simulink model "faza"  (R2025b)
settings: Solver=VariableStepAuto  StartTime=0.0  StopTime=100  MaxStep=0.01  RelTol=1e-3
values from neighbouring files (symbols this model uses):
  czas_skoku = 10    [portrety_fazowe.m]
  ksi = -5    [portrety_fazowe.m]
  omega = 2    [portrety_fazowe.m]
  skok = 0    [portrety_fazowe.m]
  x10 = tabx10(i)    [portrety_fazowe.m]
  x20 = tabx20(i)    [portrety_fazowe.m]
settings Model: Creator=mikol  LastModifiedBy=mikol

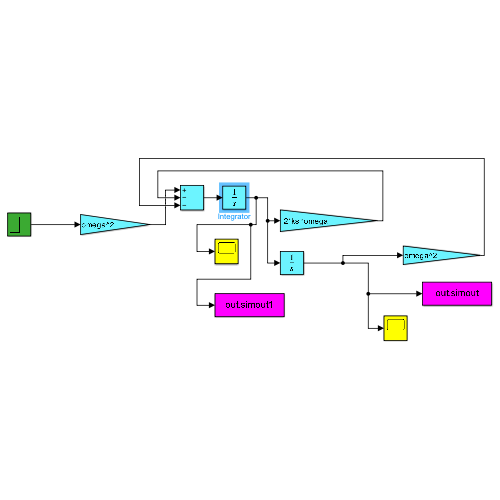
[thumbnail: Simulink's stored preview of the top-level diagram]
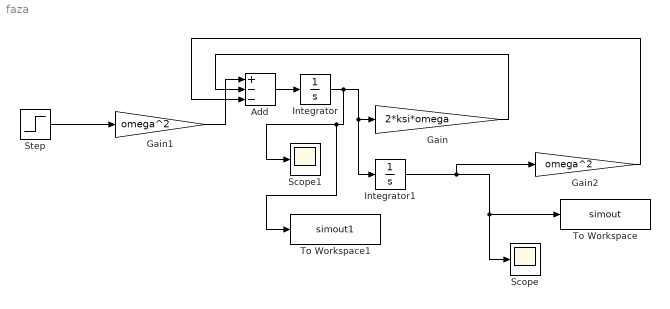
== system faza ==
  Add : Sum  Inputs=+--
  Gain : Gain  Gain=2*ksi*omega
  Gain1 : Gain  Gain=omega^2
  Gain2 : Gain  Gain=omega^2
  Integrator : Integrator  InitialCondition=x10
  Integrator1 : Integrator  InitialCondition=x20
  Scope : Scope
      settings: ActiveDisplayYMinimum=-1  ActiveDisplayYMaximum=1
  Scope1 : Scope
      settings: ActiveDisplayYMinimum=-1  ActiveDisplayYMaximum=1
  Step : Step  Time=czas_skoku  After=skok  SampleTime=0
  To Workspace : ToWorkspace  VariableName=simout  SampleTime=-1
  To Workspace1 : ToWorkspace  VariableName=simout1  SampleTime=-1
  wires:
  Integrator/1 -> To Workspace1/1, Scope1/1, Gain/1, Integrator1/1
  Integrator1/1 -> Scope/1, To Workspace/1, Gain2/1
  Step/1 -> Gain1/1
  Gain1/1 -> Add/1
  Add/1 -> Integrator/1
  Gain/1 -> Add/2
  Gain2/1 -> Add/3
